simulink model "right_arm"  (R2014b)
settings: Solver=ode45  StartTime=0.0  StopTime=10  FixedStep=1e-3  RelTol=1e-3
undefined symbols (not defined in the file or in its folder): MX28_inertia, MX28_Te, X, Y, Z
libraries: sm_lib x22, nesl_utility x11
settings Model: Creator=florent  LastModifiedBy=florent
settings DebuggingCC: IntegerOverflowMsg=none  ParameterDowncastMsg=warning  ParameterPrecisionLossMsg=none  ParameterTunabilityLossMsg=none  StateNameClashWarn=warning  IntegerSaturationMsg=none

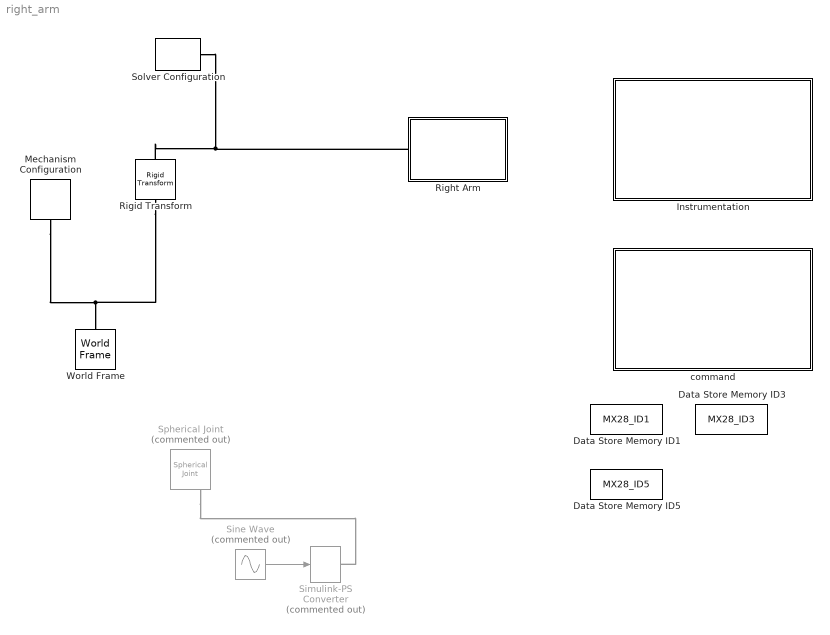
== system right_arm ==
  Data Store Memory ID1 : DataStoreMemory  DataStoreName=MX28_ID1  WriteAfterWriteMsg=error  InitialValue=MX28_default  VectorParams1D=off  OutDataTypeStr=Bus: MX28_bus
  Data Store Memory ID3 : DataStoreMemory  DataStoreName=MX28_ID3  WriteAfterWriteMsg=error  InitialValue=MX28_default  VectorParams1D=off  OutDataTypeStr=Bus: MX28_bus
  Data Store Memory ID5 : DataStoreMemory  DataStoreName=MX28_ID5  WriteAfterWriteMsg=error  InitialValue=MX28_default  VectorParams1D=off  OutDataTypeStr=Bus: MX28_bus
  Instrumentation : Subsystem
  Mechanism Configuration : sm_lib/Utilities/Mechanism Configuration  UniformGravity=Constant  GravityVector=[0 0 -9.80665]  GravityUnits=m/s^2  LinearizationDelta=0.001  BlockFunction=simmechanics.library.utilities.mechanism_configuration
  Right Arm : Subsystem
      mask init:
      | [ModelDir,~,~] = fileparts(which(gcs));
      | 
      | Block = [gcb '/Right Shoulder/Solid'];
      | STLFileName = [ModelDir filesep 'STL' filesep 'Right_shoulder.STL'];
      | if ~strcmp(get_param(Block,'ExtGeomFileName'),STLFileName)
      |     set_param(Block,'ExtGeomFileName',STLFileName);
      | end
      | 
      | Block = [gcb '/Right Upper Arm/Solid'];
      | STLFileName = [ModelDir filesep 'STL' filesep 'Right_Arm.STL'];
      | if ~strcmp(get_param(Block,'ExtGeomFileName'),STLFileName)
      |     set_param(Block,'ExtGeomFileName',STLFileName);
      | end
      | 
      | Block = [gcb '/Right Forearm/Solid'];
      | STLFileName = [ModelDir filesep 'STL' filesep 'Right_Forearm.STL'];
      | if ~strcmp(get_param(Block,'ExtGeomFileName'),STLFileName)
      |     set_param(Block,'ExtGeomFileName',STLFileName);
      | end
  Rigid Transform : sm_lib/Frames and Transforms/Rigid Transform  TranslationMethod=Cartesian  TranslationLengthUnit=m  TranslationStandardAxis=+Z  TranslationStandardOffset=0  TranslationCartesianOffset=[0 -0.001 0]  TranslationROffset=0  TranslationROffsetUnits=m  TranslationZOffset=0  TranslationZOffsetUnits=m  TranslationThetaOffset=0  TranslationThetaOffsetUnits=deg  RotationMethod=AlignedAxes  RotationAngleUnits=deg  RotationStandardAxis=+Z  RotationAngle=0  RotationArbitraryAxis=[0 0 1]  FollAlignAxisA=+Y  BaseAlignAxisA=+Z  FollAlignAxisB=+Z  BaseAlignAxisB=-X  RotationMatrix=[1 0 0; 0 1 0; 0 0 1]  BlockFunction=simmechanics.library.frames_transforms.rigid_transform
  Simulink-PS Converter : nesl_utility/Simulink-PS Converter  Commented=on  PhysicalDomain=network_engine_domain  SubClassName=ps_input  LeftPortType=input  RightPortType=output  PseudoPeriodic=off  Frequencies=[]  NoiseDistribution=none  NoiseParameters=[]  Unit=1  AffineConversion=off  InputFiltering=off  SimscapeFilterOrder=1  InputFilterTimeConstant=0.001  UdotUserProvided=1
  Sine Wave : Sin  Commented=on  Amplitude=0.1  Frequency=10  SampleTime=0
  Solver Configuration : nesl_utility/Solver Configuration  PhysicalDomain=network_engine_domain  SubClassName=solver  LeftPortType=input  RightPortType=generic  Accelerate=off  Tones=[]  Harmonics=[]  SimulateNoise=off  Profile=off  UseLocalSampling=off  EnableSwitchedLinearOptims=on  FrequencyDomain=off  UseCCode=off  RelTol=0.001  AbsTol=1e-06  MinStep=1e-09  ToWorkspace=off  DoDC=off  ResidualTolerance=1e-05  UseLocalSolver=off  LocalSolverChoice=NE_BACKWARD_EULER_ADVANCER  LocalSolverSampleTime=0.001  DoFixedCost=off  MaxNonlinIter=3  MaxModeIter=2  LinearAlgebra=Sparse  DelaysMemoryBudget=1024  AutomaticFiltering=on  FilteringTimeConstant=0.001
  Spherical Joint : sm_lib/Joints/Spherical Joint  Commented=on  SenseConstraintForce=off  SenseConstraintForceX=off  SenseConstraintForceY=off  SenseConstraintForceZ=off  SenseConstraintTorque=off  SenseConstraintTorqueX=off  SenseConstraintTorqueY=off  SenseConstraintTorqueZ=off  SenseTotalForce=off  SenseTotalForceX=off  SenseTotalForceY=off  SenseTotalForceZ=off  SenseTotalTorque=off  SenseTotalTorqueX=off  SenseTotalTorqueY=off  SenseTotalTorqueZ=off  CompositeWrenchDir=FollowerOnBase  CompositeWrenchFrame=BaseFrame  DefPosRotationMethod=None  DefPosRotationAngleUnits=deg  DefPosRotationStandardAxis=+Z  DefPosRotationAngle=0  DefPosRotationArbitraryAxis=[0 0 1]  DefPosFollAlignAxisA=+X  DefPosBaseAlignAxisA=+Y  DefPosFollAlignAxisB=+Y  DefPosBaseAlignAxisB=+Z  DefPosRotationMatrix=[1 0 0; 0 1 0; 0 0 1]  EqPosRotationMethod=None  EqPosRotationAngleUnits=deg  EqPosRotationStandardAxis=+Z  EqPosRotationAngle=0  EqPosRotationArbitraryAxis=[0 0 1]  EqPosFollAlignAxisA=+X  EqPosBaseAlignAxisA=+Y  EqPosFollAlignAxisB=+Y  EqPosBaseAlignAxisB=+Z  EqPosRotationMatrix=[1 0 0; 0 1 0; 0 0 1]  SpringStiffness=0  SpringStiffnessUnits=N*m/deg  DampingCoefficient=0  DampingCoefficientUnits=N*m/(deg/s)  ActuateTorqueX=off  ActuateTorqueY=on  ActuateTorqueZ=off  ActuateTorque=off  TorqueActuationMode=InputTorque  MotionActuationMode=ComputedMotion  ActuationFrame=BaseFrame  SensePosition=off  SenseVelocityX=off  SenseVelocityY=off  SenseVelocityZ=off  SenseVelocity=off  SenseAccelerationX=off  SenseAccelerationY=off  SenseAccelerationZ=off  SenseAcceleration=off  SenseTorqueX=off  SenseTorqueY=off  SenseTorqueZ=off  SenseTorqueForce=off  SensingFrame=BaseFrame  PositionTargetRotationMethod=ArbitraryAxis  PositionTargetRotationAngleUnits=deg  PositionTargetRotationStandardAxis=+Z  PositionTargetRotationAngle=0  PositionTargetRotationArbitraryAxis=[0 -1 0]  PositionTargetFollAlignAxisA=+X  PositionTargetBaseAlignAxisA=+Y  PositionTargetFollAlignAxisB=+Y  PositionTargetBaseAlignAxisB=+Z  PositionTargetRotationMatrix=[1 0 0; 0 1 0; 0 0 1]  PositionTargetSpecify=on  PositionTargetPriority=High  VelocityTargetValue=[0 0 0]  VelocityTargetValueUnits=deg/s  VelocityTargetSpecify=off  VelocityTargetPriority=High  VelocityTargetInFollowerFrame=on  BlockFunction=simmechanics.library.joints.spherical_joint
  World Frame : sm_lib/Frames and Transforms/World Frame  BlockFunction=simmechanics.library.frames_transforms.world_frame
  command : Subsystem
  wires:
  Sine Wave/1 -> Simulink-PS Converter/1
  connections:
  Solver Configuration/RConn1 -- Right Arm/LConn1 -- Rigid Transform/RConn1
  Mechanism Configuration/RConn1 -- Rigid Transform/LConn1 -- World Frame/RConn1
  Spherical Joint/LConn2 -- Simulink-PS Converter/RConn1

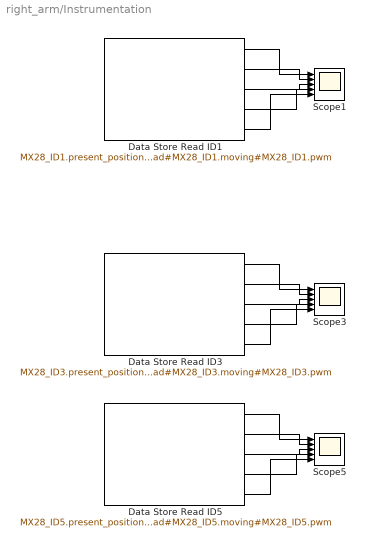
== system right_arm/Instrumentation ==
  Data Store Read ID1 : DataStoreRead  DataStoreName=MX28_ID1  SampleTime=0.001  DataStoreElements=MX28_ID1.present_position#MX28_ID1.present_speed#MX28_ID1.present_load#MX28_ID1.moving#MX28_ID1.pwm
  Data Store Read ID3 : DataStoreRead  DataStoreName=MX28_ID3  SampleTime=0.001  DataStoreElements=MX28_ID3.present_position#MX28_ID3.present_speed#MX28_ID3.present_load#MX28_ID3.moving#MX28_ID3.pwm
  Data Store Read ID5 : DataStoreRead  DataStoreName=MX28_ID5  SampleTime=0.001  DataStoreElements=MX28_ID5.present_position#MX28_ID5.present_speed#MX28_ID5.present_load#MX28_ID5.moving#MX28_ID5.pwm
  Scope1 : Scope  NumInputPorts=5
      settings: YMin=1000~-200~-500~-1~-500  YMax=3000~200~500~1~500
  Scope3 : Scope  NumInputPorts=5
      settings: YMin=-5~0~-5~-5~-5  YMax=5~650~5~5~5
  Scope5 : Scope  NumInputPorts=5
      settings: YMin=-5~0~-5~-5~-5  YMax=5~650~5~5~5  SaveName=ScopeData2
  wires:
  Data Store Read ID1/1 -> Scope1/1
  Data Store Read ID1/2 -> Scope1/2
  Data Store Read ID1/3 -> Scope1/3
  Data Store Read ID1/4 -> Scope1/4
  Data Store Read ID3/1 -> Scope3/1
  Data Store Read ID3/2 -> Scope3/2
  Data Store Read ID3/3 -> Scope3/3
  Data Store Read ID3/4 -> Scope3/4
  Data Store Read ID1/5 -> Scope1/5
  Data Store Read ID3/5 -> Scope3/5
  Data Store Read ID5/1 -> Scope5/1
  Data Store Read ID5/2 -> Scope5/2
  Data Store Read ID5/3 -> Scope5/3
  Data Store Read ID5/4 -> Scope5/4
  Data Store Read ID5/5 -> Scope5/5

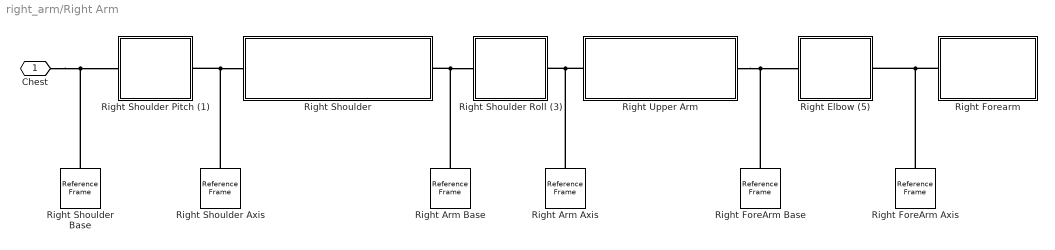
== system right_arm/Right Arm ==
  Right Arm Axis : sm_lib/Frames and Transforms/Reference Frame  BlockFunction=simmechanics.library.frames_transforms.reference_frame
  Right Arm Base : sm_lib/Frames and Transforms/Reference Frame  BlockFunction=simmechanics.library.frames_transforms.reference_frame
  Right Elbow (5) : Subsystem
  Right ForeArm Axis : sm_lib/Frames and Transforms/Reference Frame  BlockFunction=simmechanics.library.frames_transforms.reference_frame
  Right ForeArm Base : sm_lib/Frames and Transforms/Reference Frame  BlockFunction=simmechanics.library.frames_transforms.reference_frame
  Right Forearm : Subsystem
  Right Shoulder : Subsystem
  Right Shoulder Axis : sm_lib/Frames and Transforms/Reference Frame  BlockFunction=simmechanics.library.frames_transforms.reference_frame
  Right Shoulder Base : sm_lib/Frames and Transforms/Reference Frame  BlockFunction=simmechanics.library.frames_transforms.reference_frame
  Right Shoulder Pitch (1) : Subsystem
  Right Shoulder Roll (3) : Subsystem
  Right Upper Arm : Subsystem
  Chest : PMIOPort  Port=1  Side=Left
  connections:
  Chest/RConn1 -- Right Shoulder Pitch (1)/LConn1 -- Right Shoulder Base/RConn1
  Right Shoulder Axis/RConn1 -- Right Shoulder Pitch (1)/RConn1 -- Right Shoulder/LConn1
  Right Upper Arm/RConn1 -- Right Elbow (5)/LConn1 -- Right ForeArm Base/RConn1
  Right Arm Base/RConn1 -- Right Shoulder Roll (3)/LConn1 -- Right Shoulder/RConn1
  Right Arm Axis/RConn1 -- Right Shoulder Roll (3)/RConn1 -- Right Upper Arm/LConn1
  Right ForeArm Axis/RConn1 -- Right Elbow (5)/RConn1 -- Right Forearm/LConn1

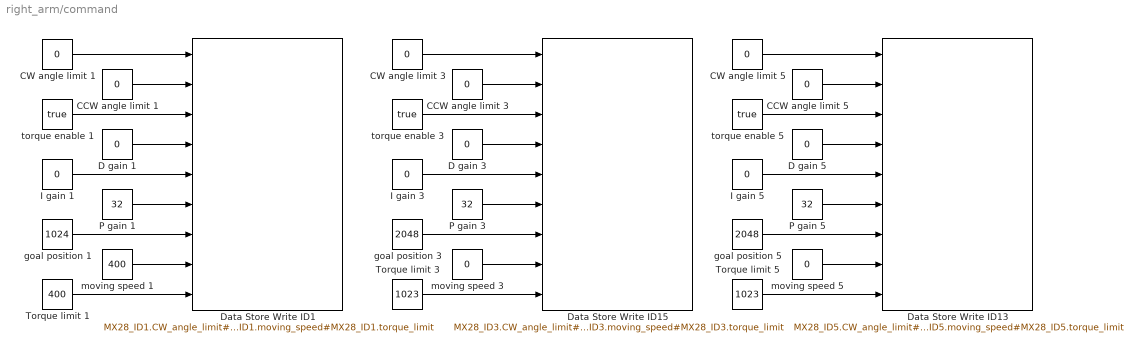
== system right_arm/command ==
  CCW angle limit 1 : Constant  Value=0  OutDataTypeStr=int16
  CCW angle limit 3 : Constant  Value=0  OutDataTypeStr=int16
  CCW angle limit 5 : Constant  Value=0  OutDataTypeStr=int16
  CW angle limit 1 : Constant  Value=0  OutDataTypeStr=int16
  CW angle limit 3 : Constant  Value=0  OutDataTypeStr=int16
  CW angle limit 5 : Constant  Value=0  OutDataTypeStr=int16
  D gain 1 : Constant  Value=0  OutDataTypeStr=uint8
  D gain 3 : Constant  Value=0  OutDataTypeStr=uint8
  D gain 5 : Constant  Value=0  OutDataTypeStr=uint8
  Data Store Write ID1 : DataStoreWrite  DataStoreName=MX28_ID1  DataStoreElements=MX28_ID1.CW_angle_limit#MX28_ID1.CCW_angle_limit#MX28_ID1.torque_enable#MX28_ID1.D_gain#MX28_ID1.I_gain#MX28_ID1.P_gain#MX28_ID1.goal_position#MX28_ID1.moving_speed#MX28_ID1.torque_limit
  Data Store Write ID13 : DataStoreWrite  DataStoreName=MX28_ID5  DataStoreElements=MX28_ID5.CW_angle_limit#MX28_ID5.CCW_angle_limit#MX28_ID5.torque_enable#MX28_ID5.D_gain#MX28_ID5.I_gain#MX28_ID5.P_gain#MX28_ID5.goal_position#MX28_ID5.moving_speed#MX28_ID5.torque_limit
  Data Store Write ID15 : DataStoreWrite  DataStoreName=MX28_ID3  DataStoreElements=MX28_ID3.CW_angle_limit#MX28_ID3.CCW_angle_limit#MX28_ID3.torque_enable#MX28_ID3.D_gain#MX28_ID3.I_gain#MX28_ID3.P_gain#MX28_ID3.goal_position#MX28_ID3.moving_speed#MX28_ID3.torque_limit
  I gain 1 : Constant  Value=0  OutDataTypeStr=uint8
  I gain 3 : Constant  Value=0  OutDataTypeStr=uint8
  I gain 5 : Constant  Value=0  OutDataTypeStr=uint8
  P gain 1 : Constant  Value=32  OutDataTypeStr=uint8
  P gain 3 : Constant  Value=32  OutDataTypeStr=uint8
  P gain 5 : Constant  Value=32  OutDataTypeStr=uint8
  Torque limit 1 : Constant  Value=400  OutDataTypeStr=int16
  Torque limit 3 : Constant  Value=1023  OutDataTypeStr=int16
  Torque limit 5 : Constant  Value=1023  OutDataTypeStr=int16
  goal position 1 : Constant  Value=1024  OutDataTypeStr=int16
  goal position 3 : Constant  Value=2048  OutDataTypeStr=int16
  goal position 5 : Constant  Value=2048  OutDataTypeStr=int16
  moving speed 1 : Constant  Value=400  OutDataTypeStr=int16
  moving speed 3 : Constant  Value=0  OutDataTypeStr=int16
  moving speed 5 : Constant  Value=0  OutDataTypeStr=int16
  torque enable 1 : Constant  Value=true  OutDataTypeStr=boolean
  torque enable 3 : Constant  Value=true  OutDataTypeStr=boolean
  torque enable 5 : Constant  Value=true  OutDataTypeStr=boolean
  wires:
  Torque limit 1/1 -> Data Store Write ID1/9
  moving speed 1/1 -> Data Store Write ID1/8
  goal position 1/1 -> Data Store Write ID1/7
  P gain 1/1 -> Data Store Write ID1/6
  I gain 1/1 -> Data Store Write ID1/5
  D gain 1/1 -> Data Store Write ID1/4
  torque enable 1/1 -> Data Store Write ID1/3
  CW angle limit 1/1 -> Data Store Write ID1/1
  CCW angle limit 1/1 -> Data Store Write ID1/2
  Torque limit 3/1 -> Data Store Write ID15/9
  moving speed 3/1 -> Data Store Write ID15/8
  goal position 3/1 -> Data Store Write ID15/7
  P gain 3/1 -> Data Store Write ID15/6
  I gain 3/1 -> Data Store Write ID15/5
  D gain 3/1 -> Data Store Write ID15/4
  torque enable 3/1 -> Data Store Write ID15/3
  CCW angle limit 3/1 -> Data Store Write ID15/2
  CW angle limit 3/1 -> Data Store Write ID15/1
  Torque limit 5/1 -> Data Store Write ID13/9
  moving speed 5/1 -> Data Store Write ID13/8
  goal position 5/1 -> Data Store Write ID13/7
  P gain 5/1 -> Data Store Write ID13/6
  I gain 5/1 -> Data Store Write ID13/5
  D gain 5/1 -> Data Store Write ID13/4
  torque enable 5/1 -> Data Store Write ID13/3
  CW angle limit 5/1 -> Data Store Write ID13/1
  CCW angle limit 5/1 -> Data Store Write ID13/2

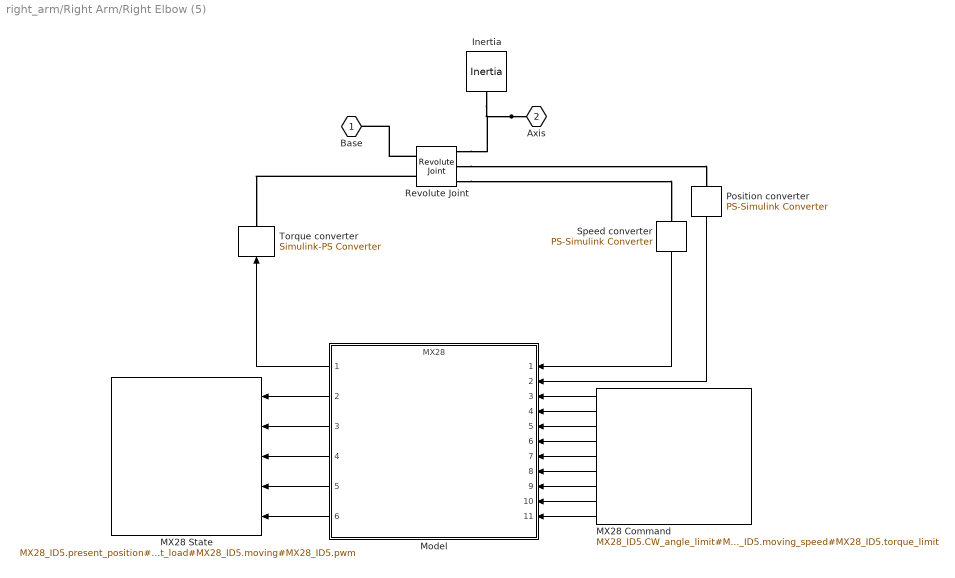
== system right_arm/Right Arm/Right Elbow (5) ==
  Inertia : sm_lib/Body Elements/Inertia  InertiaType=Custom  Mass=1  MassUnits=g  CenterOfMass=[0 0 0]  CenterOfMassUnits=m  MomentsOfInertia=[0 0 MX28_inertia]  MomentsOfInertiaUnits=kg*m^2  ProductsOfInertia=[0 0 0]  ProductsOfInertiaUnits=kg*m^2  BlockFunction=simmechanics.library.body_elements.inertia
  MX28 Command : DataStoreRead  DataStoreName=MX28_ID5  SampleTime=MX28_Te  DataStoreElements=MX28_ID5.CW_angle_limit#MX28_ID5.CCW_angle_limit#MX28_ID5.torque_enable#MX28_ID5.D_gain#MX28_ID5.I_gain#MX28_ID5.P_gain#MX28_ID5.goal_position#MX28_ID5.moving_speed#MX28_ID5.torque_limit
  MX28 State : DataStoreWrite  DataStoreName=MX28_ID5  DataStoreElements=MX28_ID5.present_position#MX28_ID5.present_speed#MX28_ID5.present_load#MX28_ID5.moving#MX28_ID5.pwm
  Model : ModelReference  ModelNameDialog=MX28.slx  SimulationMode=Normal  ModelReferenceVersion=1.66  CopyOfModelName=MX28.slx  DefaultDataLogging=on
  Position converter : nesl_utility/PS-Simulink Converter  PhysicalDomain=network_engine_domain  SubClassName=ps_output  LeftPortType=input  RightPortType=output  PseudoPeriodic=off  Frequencies=[]  Unit=rad  AffineConversion=off
  Revolute Joint : sm_lib/Joints/Revolute Joint  SenseConstraintForce=off  SenseConstraintForceX=off  SenseConstraintForceY=off  SenseConstraintForceZ=off  SenseConstraintTorque=off  SenseConstraintTorqueX=off  SenseConstraintTorqueY=off  SenseConstraintTorqueZ=off  SenseTotalForce=off  SenseTotalForceX=off  SenseTotalForceY=off  SenseTotalForceZ=off  SenseTotalTorque=off  SenseTotalTorqueX=off  SenseTotalTorqueY=off  SenseTotalTorqueZ=off  CompositeWrenchDir=FollowerOnBase  CompositeWrenchFrame=BaseFrame  EquilibriumPosition=0  EquilibriumPositionUnits=deg  SpringStiffness=0  SpringStiffnessUnits=N*m/deg  DampingCoefficient=MX28_lub_friction  DampingCoefficientUnits=N*m/(rad/s)  TorqueActuationMode=InputTorque  MotionActuationMode=ComputedMotion  SensePosition=on  SenseVelocity=on  SenseAcceleration=off  SenseTorqueForce=off  PositionTargetValue=MX28_init_position  PositionTargetValueUnits=rad  PositionTargetSpecify=on  PositionTargetPriority=High  VelocityTargetValue=MX28_init_speed  VelocityTargetValueUnits=rad/s  VelocityTargetSpecify=on  VelocityTargetPriority=High  BlockFunction=simmechanics.library.joints.revolute_joint
  Speed converter : nesl_utility/PS-Simulink Converter  PhysicalDomain=network_engine_domain  SubClassName=ps_output  LeftPortType=input  RightPortType=output  PseudoPeriodic=off  Frequencies=[]  Unit=rad/s  AffineConversion=off
  Torque converter : nesl_utility/Simulink-PS Converter  PhysicalDomain=network_engine_domain  SubClassName=ps_input  LeftPortType=input  RightPortType=output  PseudoPeriodic=off  Frequencies=[]  NoiseDistribution=none  NoiseParameters=[]  Unit=N*m  AffineConversion=off  InputFiltering=off  SimscapeFilterOrder=1  InputFilterTimeConstant=0.001  UdotUserProvided=1
  Base : PMIOPort  Port=1  Side=Left
  Axis : PMIOPort  Port=2  Side=Right
  wires:
  Model/4 -> MX28 State/3
  Model/2 -> MX28 State/1
  Model/5 -> MX28 State/4
  Model/3 -> MX28 State/2
  MX28 Command/3 -> Model/5
  MX28 Command/6 -> Model/8
  MX28 Command/4 -> Model/6
  MX28 Command/5 -> Model/7
  MX28 Command/7 -> Model/9
  MX28 Command/2 -> Model/4
  MX28 Command/1 -> Model/3
  Speed converter/1 -> Model/1
  Position converter/1 -> Model/2
  Model/1 -> Torque converter/1
  Model/6 -> MX28 State/5
  MX28 Command/8 -> Model/10
  MX28 Command/9 -> Model/11
  connections:
  Axis/RConn1 -- Revolute Joint/RConn1 -- Inertia/RConn1
  Revolute Joint/RConn3 -- Speed converter/LConn1
  Revolute Joint/RConn2 -- Position converter/LConn1
  Revolute Joint/LConn2 -- Torque converter/RConn1
  Revolute Joint/LConn1 -- Base/RConn1

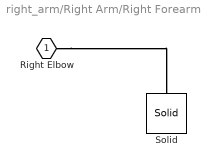
== system right_arm/Right Arm/Right Forearm ==
  Solid : sm_lib/Body Elements/Solid  InertiaType=Custom  Mass=62.79  MassUnits=g  CenterOfMass=[12.76 43.34 -15.75]  CenterOfMassUnits=mm  MomentsOfInertia=[94510 21923 95153]  MomentsOfInertiaUnits=g*mm^2  ProductsOfInertia=[1625 -659.23 8489]  ProductsOfInertiaUnits=g*mm^2  DensityBased=on  Density=1000  DensityUnits=kg/(m^3)  GraphicType=FromGeometry  MarkerShape=Sphere  MarkerSize=10  MarkerSizeUnits=m  GraphicVisPropType=SimpleVisualProperties  GraphicDiffuseColor=[0.5 0.5 0.5]  GraphicSpecularColor=[0.5 0.5 0.5 1.0]  GraphicAmbientColor=[0.15 0.15 0.15 1.0]  GraphicEmissiveColor=[0.0 0.0 0.0 1.0]  GraphicShininess=75  GraphicOpacity=1.0  GeometryShape=FromFile  RectangleSize=[1 1]  RectangleSizeUnits=m  BrickDimensions=[1 1 1]  BrickDimensionUnits=m  CylinderRadius=1  CylinderRadiusUnits=m  CylinderLength=1  CylinderLengthUnits=m  SphereRadius=1  SphereRadiusUnits=m  EllipsoidRadii=[1 1 1]  EllipsoidRadiiUnits=m  ExtrusionCrossSection=[1 1; -1 1; -1 -1; 1 -1]  ExtrusionCrossSectionUnits=m  ExtrusionLength=1  ExtrusionLengthUnits=m  PolygonNumSides=3  PolygonOuterRadius=1  PolygonOuterRadiusUnits=m  ExtGeomFileType=STL  ExtGeomFileName=D:\Ker Lann\systemes\darwin\kinematics\STL\Right_Forearm.STL  ExtGeomFileUnits=mm  RevolutionCrossSection=[1 1; 1 -1; 2 -1; 2 1]  RevolutionCrossSectionUnits=m  RevolutionExtent=Full  RevolutionAngle=180  RevolutionAngleUnits=deg  BlockFunction=simmechanics.library.body_elements.solid
  Right Elbow : PMIOPort  Port=1  Side=Left
  connections:
  Right Elbow/RConn1 -- Solid/RConn1

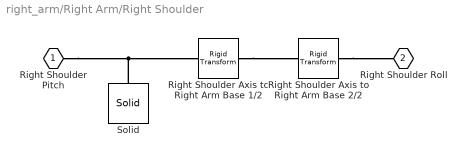
== system right_arm/Right Arm/Right Shoulder ==
  Right Shoulder Axis to Right Arm Base 1/2 : sm_lib/Frames and Transforms/Rigid Transform  TranslationMethod=Cartesian  TranslationLengthUnit=mm  TranslationStandardAxis=+Z  TranslationStandardOffset=0  TranslationCartesianOffset=[-23.65 16 21.35]  TranslationROffset=0  TranslationROffsetUnits=m  TranslationZOffset=0  TranslationZOffsetUnits=m  TranslationThetaOffset=0  TranslationThetaOffsetUnits=deg  RotationMethod=StandardAxis  RotationAngleUnits=deg  RotationStandardAxis=+Y  RotationAngle=270  RotationArbitraryAxis=[0 0 1]  FollAlignAxisA=+X  BaseAlignAxisA=+Y  FollAlignAxisB=+Y  BaseAlignAxisB=+Z  RotationMatrix=[1 0 0; 0 1 0; 0 0 1]  BlockFunction=simmechanics.library.frames_transforms.rigid_transform
  Right Shoulder Axis to Right Arm Base 2/2 : sm_lib/Frames and Transforms/Rigid Transform  TranslationMethod=None  TranslationLengthUnit=mm  TranslationStandardAxis=+Z  TranslationStandardOffset=0  TranslationCartesianOffset=[-23.65 16 21.35]  TranslationROffset=0  TranslationROffsetUnits=m  TranslationZOffset=0  TranslationZOffsetUnits=m  TranslationThetaOffset=0  TranslationThetaOffsetUnits=deg  RotationMethod=StandardAxis  RotationAngleUnits=deg  RotationStandardAxis=+Z  RotationAngle=+135  RotationArbitraryAxis=[0 0 1]  FollAlignAxisA=+X  BaseAlignAxisA=+Y  FollAlignAxisB=+Y  BaseAlignAxisB=+Z  RotationMatrix=[1 0 0; 0 1 0; 0 0 1]  BlockFunction=simmechanics.library.frames_transforms.rigid_transform
  Solid : sm_lib/Body Elements/Solid  InertiaType=Custom  Mass=34.03  MassUnits=g  CenterOfMass=[-4.16 5.98 7.64]  CenterOfMassUnits=mm  MomentsOfInertia=[7413 12768 11409]  MomentsOfInertiaUnits=g*mm^2  ProductsOfInertia=[2455 -1943 -1420]  ProductsOfInertiaUnits=g*mm^2  DensityBased=on  Density=1000  DensityUnits=kg/(m^3)  GraphicType=FromGeometry  MarkerShape=Sphere  MarkerSize=10  MarkerSizeUnits=m  GraphicVisPropType=SimpleVisualProperties  GraphicDiffuseColor=[0.5 0.5 0.5]  GraphicSpecularColor=[0.5 0.5 0.5 1.0]  GraphicAmbientColor=[0.15 0.15 0.15 1.0]  GraphicEmissiveColor=[0.0 0.0 0.0 1.0]  GraphicShininess=75  GraphicOpacity=1.0  GeometryShape=FromFile  RectangleSize=[1 1]  RectangleSizeUnits=m  BrickDimensions=[1 1 1]  BrickDimensionUnits=m  CylinderRadius=1  CylinderRadiusUnits=m  CylinderLength=1  CylinderLengthUnits=m  SphereRadius=1  SphereRadiusUnits=m  EllipsoidRadii=[1 1 1]  EllipsoidRadiiUnits=m  ExtrusionCrossSection=[1 1; -1 1; -1 -1; 1 -1]  ExtrusionCrossSectionUnits=m  ExtrusionLength=1  ExtrusionLengthUnits=m  PolygonNumSides=3  PolygonOuterRadius=1  PolygonOuterRadiusUnits=m  ExtGeomFileType=STL  ExtGeomFileName=D:\Ker Lann\systemes\darwin\kinematics\STL\Right_shoulder.STL  ExtGeomFileUnits=mm  RevolutionCrossSection=[1 1; 1 -1; 2 -1; 2 1]  RevolutionCrossSectionUnits=m  RevolutionExtent=Full  RevolutionAngle=180  RevolutionAngleUnits=deg  BlockFunction=simmechanics.library.body_elements.solid
  Right Shoulder Pitch : PMIOPort  Port=1  Side=Left
  Right Shoulder Roll : PMIOPort  Port=2  Side=Right
  connections:
  Solid/RConn1 -- Right Shoulder Axis to Right Arm Base 1/2/LConn1 -- Right Shoulder Pitch/RConn1
  Right Shoulder Axis to Right Arm Base 2/2/RConn1 -- Right Shoulder Roll/RConn1
  Right Shoulder Axis to Right Arm Base 1/2/RConn1 -- Right Shoulder Axis to Right Arm Base 2/2/LConn1

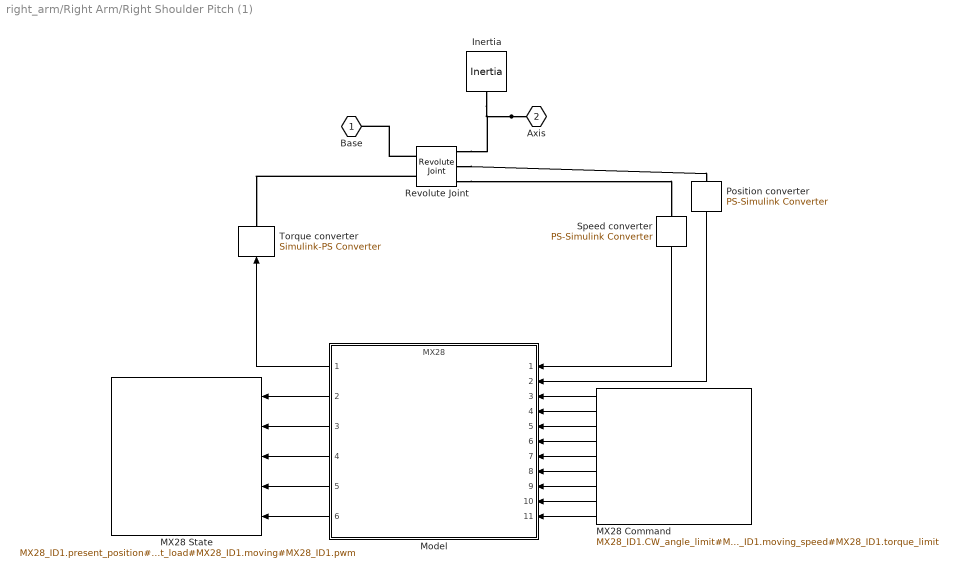
== system right_arm/Right Arm/Right Shoulder Pitch (1) ==
  Inertia : sm_lib/Body Elements/Inertia  InertiaType=Custom  Mass=1  MassUnits=g  CenterOfMass=[0 0 0]  CenterOfMassUnits=m  MomentsOfInertia=[0 0 MX28_inertia]  MomentsOfInertiaUnits=kg*m^2  ProductsOfInertia=[0 0 0]  ProductsOfInertiaUnits=kg*m^2  BlockFunction=simmechanics.library.body_elements.inertia
  MX28 Command : DataStoreRead  DataStoreName=MX28_ID1  SampleTime=MX28_Te  DataStoreElements=MX28_ID1.CW_angle_limit#MX28_ID1.CCW_angle_limit#MX28_ID1.torque_enable#MX28_ID1.D_gain#MX28_ID1.I_gain#MX28_ID1.P_gain#MX28_ID1.goal_position#MX28_ID1.moving_speed#MX28_ID1.torque_limit
  MX28 State : DataStoreWrite  DataStoreName=MX28_ID1  DataStoreElements=MX28_ID1.present_position#MX28_ID1.present_speed#MX28_ID1.present_load#MX28_ID1.moving#MX28_ID1.pwm
  Model : ModelReference  ModelNameDialog=MX28.slx  SimulationMode=Normal  ModelReferenceVersion=1.66  CopyOfModelName=MX28.slx  DefaultDataLogging=on
  Position converter : nesl_utility/PS-Simulink Converter  PhysicalDomain=network_engine_domain  SubClassName=ps_output  LeftPortType=input  RightPortType=output  PseudoPeriodic=off  Frequencies=[]  Unit=rad  AffineConversion=off
  Revolute Joint : sm_lib/Joints/Revolute Joint  SenseConstraintForce=off  SenseConstraintForceX=off  SenseConstraintForceY=off  SenseConstraintForceZ=off  SenseConstraintTorque=off  SenseConstraintTorqueX=off  SenseConstraintTorqueY=off  SenseConstraintTorqueZ=off  SenseTotalForce=off  SenseTotalForceX=off  SenseTotalForceY=off  SenseTotalForceZ=off  SenseTotalTorque=off  SenseTotalTorqueX=off  SenseTotalTorqueY=off  SenseTotalTorqueZ=off  CompositeWrenchDir=FollowerOnBase  CompositeWrenchFrame=BaseFrame  EquilibriumPosition=0  EquilibriumPositionUnits=deg  SpringStiffness=0  SpringStiffnessUnits=N*m/deg  DampingCoefficient=MX28_lub_friction  DampingCoefficientUnits=N*m/(rad/s)  TorqueActuationMode=InputTorque  MotionActuationMode=ComputedMotion  SensePosition=on  SenseVelocity=on  SenseAcceleration=off  SenseTorqueForce=off  PositionTargetValue=MX28_init_position  PositionTargetValueUnits=rad  PositionTargetSpecify=on  PositionTargetPriority=High  VelocityTargetValue=MX28_init_speed  VelocityTargetValueUnits=rad/s  VelocityTargetSpecify=on  VelocityTargetPriority=High  BlockFunction=simmechanics.library.joints.revolute_joint
  Speed converter : nesl_utility/PS-Simulink Converter  PhysicalDomain=network_engine_domain  SubClassName=ps_output  LeftPortType=input  RightPortType=output  PseudoPeriodic=off  Frequencies=[]  Unit=rad/s  AffineConversion=off
  Torque converter : nesl_utility/Simulink-PS Converter  PhysicalDomain=network_engine_domain  SubClassName=ps_input  LeftPortType=input  RightPortType=output  PseudoPeriodic=off  Frequencies=[]  NoiseDistribution=none  NoiseParameters=[]  Unit=N*m  AffineConversion=off  InputFiltering=off  SimscapeFilterOrder=1  InputFilterTimeConstant=0.001  UdotUserProvided=1
  Base : PMIOPort  Port=1  Side=Left
  Axis : PMIOPort  Port=2  Side=Right
  wires:
  Model/4 -> MX28 State/3
  Model/2 -> MX28 State/1
  Model/5 -> MX28 State/4
  Model/3 -> MX28 State/2
  MX28 Command/3 -> Model/5
  MX28 Command/6 -> Model/8
  MX28 Command/4 -> Model/6
  MX28 Command/5 -> Model/7
  MX28 Command/7 -> Model/9
  MX28 Command/2 -> Model/4
  MX28 Command/1 -> Model/3
  Speed converter/1 -> Model/1
  Position converter/1 -> Model/2
  Model/1 -> Torque converter/1
  Model/6 -> MX28 State/5
  MX28 Command/8 -> Model/10
  MX28 Command/9 -> Model/11
  connections:
  Axis/RConn1 -- Revolute Joint/RConn1 -- Inertia/RConn1
  Revolute Joint/LConn1 -- Base/RConn1
  Revolute Joint/RConn3 -- Speed converter/LConn1
  Revolute Joint/RConn2 -- Position converter/LConn1
  Revolute Joint/LConn2 -- Torque converter/RConn1

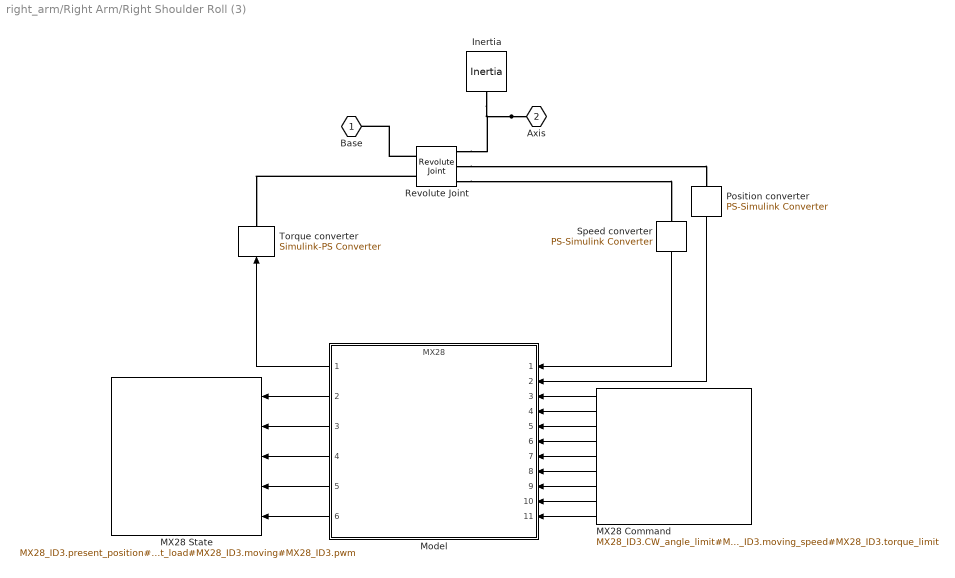
== system right_arm/Right Arm/Right Shoulder Roll (3) ==
  Inertia : sm_lib/Body Elements/Inertia  InertiaType=Custom  Mass=1  MassUnits=g  CenterOfMass=[0 0 0]  CenterOfMassUnits=m  MomentsOfInertia=[0 0 MX28_inertia]  MomentsOfInertiaUnits=kg*m^2  ProductsOfInertia=[0 0 0]  ProductsOfInertiaUnits=kg*m^2  BlockFunction=simmechanics.library.body_elements.inertia
  MX28 Command : DataStoreRead  DataStoreName=MX28_ID3  SampleTime=MX28_Te  DataStoreElements=MX28_ID3.CW_angle_limit#MX28_ID3.CCW_angle_limit#MX28_ID3.torque_enable#MX28_ID3.D_gain#MX28_ID3.I_gain#MX28_ID3.P_gain#MX28_ID3.goal_position#MX28_ID3.moving_speed#MX28_ID3.torque_limit
  MX28 State : DataStoreWrite  DataStoreName=MX28_ID3  DataStoreElements=MX28_ID3.present_position#MX28_ID3.present_speed#MX28_ID3.present_load#MX28_ID3.moving#MX28_ID3.pwm
  Model : ModelReference  ModelNameDialog=MX28.slx  SimulationMode=Normal  ModelReferenceVersion=1.66  CopyOfModelName=MX28.slx  DefaultDataLogging=on
  Position converter : nesl_utility/PS-Simulink Converter  PhysicalDomain=network_engine_domain  SubClassName=ps_output  LeftPortType=input  RightPortType=output  PseudoPeriodic=off  Frequencies=[]  Unit=rad  AffineConversion=off
  Revolute Joint : sm_lib/Joints/Revolute Joint  SenseConstraintForce=off  SenseConstraintForceX=off  SenseConstraintForceY=off  SenseConstraintForceZ=off  SenseConstraintTorque=off  SenseConstraintTorqueX=off  SenseConstraintTorqueY=off  SenseConstraintTorqueZ=off  SenseTotalForce=off  SenseTotalForceX=off  SenseTotalForceY=off  SenseTotalForceZ=off  SenseTotalTorque=off  SenseTotalTorqueX=off  SenseTotalTorqueY=off  SenseTotalTorqueZ=off  CompositeWrenchDir=FollowerOnBase  CompositeWrenchFrame=BaseFrame  EquilibriumPosition=0  EquilibriumPositionUnits=deg  SpringStiffness=0  SpringStiffnessUnits=N*m/deg  DampingCoefficient=MX28_lub_friction  DampingCoefficientUnits=N*m/(rad/s)  TorqueActuationMode=InputTorque  MotionActuationMode=ComputedMotion  SensePosition=on  SenseVelocity=on  SenseAcceleration=off  SenseTorqueForce=off  PositionTargetValue=MX28_init_position  PositionTargetValueUnits=rad  PositionTargetSpecify=on  PositionTargetPriority=High  VelocityTargetValue=MX28_init_speed  VelocityTargetValueUnits=rad/s  VelocityTargetSpecify=on  VelocityTargetPriority=High  BlockFunction=simmechanics.library.joints.revolute_joint
  Speed converter : nesl_utility/PS-Simulink Converter  PhysicalDomain=network_engine_domain  SubClassName=ps_output  LeftPortType=input  RightPortType=output  PseudoPeriodic=off  Frequencies=[]  Unit=rad/s  AffineConversion=off
  Torque converter : nesl_utility/Simulink-PS Converter  PhysicalDomain=network_engine_domain  SubClassName=ps_input  LeftPortType=input  RightPortType=output  PseudoPeriodic=off  Frequencies=[]  NoiseDistribution=none  NoiseParameters=[]  Unit=N*m  AffineConversion=off  InputFiltering=off  SimscapeFilterOrder=1  InputFilterTimeConstant=0.001  UdotUserProvided=1
  Base : PMIOPort  Port=1  Side=Left
  Axis : PMIOPort  Port=2  Side=Right
  wires:
  Model/4 -> MX28 State/3
  Model/2 -> MX28 State/1
  Model/5 -> MX28 State/4
  Model/3 -> MX28 State/2
  MX28 Command/3 -> Model/5
  MX28 Command/6 -> Model/8
  MX28 Command/4 -> Model/6
  MX28 Command/5 -> Model/7
  MX28 Command/7 -> Model/9
  MX28 Command/2 -> Model/4
  MX28 Command/1 -> Model/3
  Speed converter/1 -> Model/1
  Position converter/1 -> Model/2
  Model/1 -> Torque converter/1
  Model/6 -> MX28 State/5
  MX28 Command/8 -> Model/10
  MX28 Command/9 -> Model/11
  connections:
  Axis/RConn1 -- Revolute Joint/RConn1 -- Inertia/RConn1
  Revolute Joint/RConn3 -- Speed converter/LConn1
  Revolute Joint/RConn2 -- Position converter/LConn1
  Revolute Joint/LConn2 -- Torque converter/RConn1
  Revolute Joint/LConn1 -- Base/RConn1

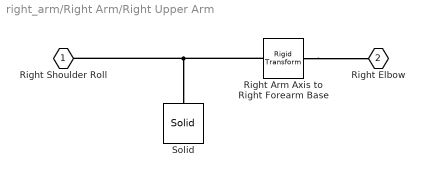
== system right_arm/Right Arm/Right Upper Arm ==
  Right Arm Axis to Right Forearm Base : sm_lib/Frames and Transforms/Rigid Transform  TranslationMethod=Cartesian  TranslationLengthUnit=mm  TranslationStandardAxis=+Z  TranslationStandardOffset=0  TranslationCartesianOffset=[23.9 60 -7.9]  TranslationROffset=0  TranslationROffsetUnits=m  TranslationZOffset=0  TranslationZOffsetUnits=m  TranslationThetaOffset=0  TranslationThetaOffsetUnits=deg  RotationMethod=AlignedAxes  RotationAngleUnits=deg  RotationStandardAxis=+Z  RotationAngle=0  RotationArbitraryAxis=[0 0 1]  FollAlignAxisA=+X  BaseAlignAxisA=-Y  FollAlignAxisB=+Z  BaseAlignAxisB=+X  RotationMatrix=[1 0 0; 0 1 0; 0 0 1]  BlockFunction=simmechanics.library.frames_transforms.rigid_transform
  Solid : sm_lib/Body Elements/Solid  InertiaType=Custom  Mass=164.27  MassUnits=g  CenterOfMass=[0.09 35.32 -22.36]  CenterOfMassUnits=mm  MomentsOfInertia=[10985 7003 10316]  MomentsOfInertiaUnits=g*mm^2  ProductsOfInertia=[1167 -369 -1558]  ProductsOfInertiaUnits=g*mm^2  DensityBased=on  Density=1000  DensityUnits=kg/(m^3)  GraphicType=FromGeometry  MarkerShape=Sphere  MarkerSize=10  MarkerSizeUnits=m  GraphicVisPropType=SimpleVisualProperties  GraphicDiffuseColor=[0.5 0.5 0.5]  GraphicSpecularColor=[0.5 0.5 0.5 1.0]  GraphicAmbientColor=[0.15 0.15 0.15 1.0]  GraphicEmissiveColor=[0.0 0.0 0.0 1.0]  GraphicShininess=75  GraphicOpacity=1.0  GeometryShape=FromFile  RectangleSize=[1 1]  RectangleSizeUnits=m  BrickDimensions=[1 1 1]  BrickDimensionUnits=mm  CylinderRadius=1  CylinderRadiusUnits=m  CylinderLength=1  CylinderLengthUnits=m  SphereRadius=1  SphereRadiusUnits=m  EllipsoidRadii=[1 1 1]  EllipsoidRadiiUnits=m  ExtrusionCrossSection=[1 1; -1 1; -1 -1; 1 -1]  ExtrusionCrossSectionUnits=m  ExtrusionLength=1  ExtrusionLengthUnits=m  PolygonNumSides=3  PolygonOuterRadius=1  PolygonOuterRadiusUnits=m  ExtGeomFileType=STL  ExtGeomFileName=D:\Ker Lann\systemes\darwin\kinematics\STL\Right_Arm.STL  ExtGeomFileUnits=mm  RevolutionCrossSection=[1 1; 1 -1; 2 -1; 2 1]  RevolutionCrossSectionUnits=m  RevolutionExtent=Full  RevolutionAngle=180  RevolutionAngleUnits=deg  BlockFunction=simmechanics.library.body_elements.solid
  Right Shoulder Roll : PMIOPort  Port=1  Side=Left
  Right Elbow : PMIOPort  Port=2  Side=Right
  connections:
  Right Arm Axis to Right Forearm Base/LConn1 -- Right Shoulder Roll/RConn1 -- Solid/RConn1
  Right Arm Axis to Right Forearm Base/RConn1 -- Right Elbow/RConn1
